simulink model "MPS_device_passive"  (R2018b)
settings: Solver=ode4  StartTime=0  StopTime=300  FixedStep=0.02  MaxStep=0.02  RelTol=1e-3  EnableMultiTasking=on
InitFcn:
  | %SSModel_calc
undefined symbols (not defined in the file): body, CentralPTOPreload, constraint, L, ML1Preload, ML2Preload, ML3Preload, ML4Preload, ML5Preload, ML6Preload, ML7Preload, ML8Preload, mrelative, pto, PTOrotation, SidePTO1Preload, SidePTO2Preload, SidePTO3Preload, SidePTO4Preload, simu, waves, X, Y, Z
libraries: nesl_utility x580, sm_lib x317, vrlib x72, WECSim_Lib x36
(part 19 of 27)

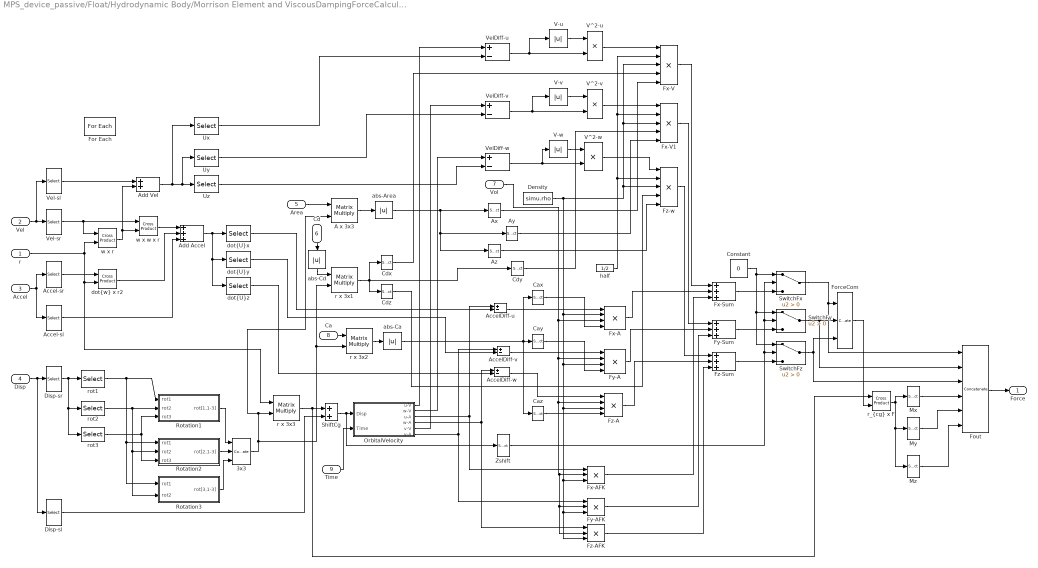
== system MPS_device_passive/Float/Hydrodynamic Body/Morrison Element and ViscousDampingForceCalculation/Morrison Element Variant Subsystem/Morrison Element On/Regular Wave Morison Force/MorrisonElements ==
  r : Inport  Partition=on  PartitionDimension=1  PartitionWidth=1  PartitionOffset=0
  Vel : Inport  Port=2
  Accel : Inport  Port=3
  Disp : Inport  Port=4
  Area : Inport  Port=5  Partition=on  PartitionDimension=1  PartitionWidth=1  PartitionOffset=0
  Cd : Inport  Port=6  Partition=on  PartitionDimension=1  PartitionWidth=1  PartitionOffset=0
  Vol : Inport  Port=7  Partition=on  PartitionDimension=1  PartitionWidth=1  PartitionOffset=0
  Ca : Inport  Port=8  Partition=on  PartitionDimension=1  PartitionWidth=1  PartitionOffset=0
  Time : Inport  Port=9
  3x3 : Concatenate  NumInputs=3  Mode=Multidimensional array
  A x 3x3 : Product  Multiplication=Matrix(*)
  Accel-sl : Selector  InputPortWidth=6  IndexOptions=Index vector (dialog)  Indices=[1 2 3]  OutputSizes=1
  Accel-sr : Selector  InputPortWidth=6  IndexOptions=Index vector (dialog)  Indices=[4 5 6]  OutputSizes=1
  AccelDiff-u : Sum  Inputs=+-
  AccelDiff-v : Sum  Inputs=+-
  AccelDiff-w : Sum  Inputs=+-
  Add Accel : Sum  Inputs=+++
  Add Vel : Sum
  Ax : Selector  InputPortWidth=3  IndexOptions=Index vector (dialog)  Indices=[1]  OutputSizes=1
  Ay : Selector  InputPortWidth=3  IndexOptions=Index vector (dialog)  Indices=[2]  OutputSizes=1
  Az : Selector  InputPortWidth=3  IndexOptions=Index vector (dialog)  Indices=[3]  OutputSizes=1
  Cax : Selector  InputPortWidth=3  IndexOptions=Index vector (dialog)  Indices=[1]  OutputSizes=1
  Cay : Selector  InputPortWidth=3  IndexOptions=Index vector (dialog)  Indices=[2]  OutputSizes=1
  Caz : Selector  InputPortWidth=3  IndexOptions=Index vector (dialog)  Indices=[3]  OutputSizes=1
  Cdx : Selector  InputPortWidth=3  IndexOptions=Index vector (dialog)  Indices=[1]  OutputSizes=1
  Cdy : Selector  InputPortWidth=3  IndexOptions=Index vector (dialog)  Indices=[2]  OutputSizes=1
  Cdz : Selector  InputPortWidth=3  IndexOptions=Index vector (dialog)  Indices=[3]  OutputSizes=1
  Constant : Constant  Value=0
  Density : Constant  Value=simu.rho
  Disp-sl : Selector  InputPortWidth=6  IndexOptions=Index vector (dialog)  Indices=[1 2 3]  OutputSizes=1
  Disp-sr : Selector  InputPortWidth=6  IndexOptions=Index vector (dialog)  Indices=[4 5 6]  OutputSizes=1
  For Each : ForEach  DisableCoverage=on  IndexMode=One-based
  ForceCom : Concatenate  NumInputs=3  ConcatenateDimension=2
  Fout : Concatenate  NumInputs=6  Mode=Multidimensional array  ConcatenateDimension=2
  Fx-A : Product  Inputs=4
  Fx-AFK : Product  Inputs=3
  Fx-Sum : Sum  Inputs=+++
  Fx-V : Product  Inputs=5
  Fx-V1 : Product  Inputs=5
  Fy-A : Product  Inputs=4
  Fy-AFK : Product  Inputs=3
  Fy-Sum : Sum  Inputs=+++
  Fz-A : Product  Inputs=4
  Fz-AFK : Product  Inputs=3
  Fz-Sum : Sum  Inputs=+++
  Fz-w : Product  Inputs=5
  Mx : Selector  InputPortWidth=3  IndexOptions=Index vector (dialog)  Indices=[1]  OutputSizes=1
  My : Selector  InputPortWidth=3  IndexOptions=Index vector (dialog)  Indices=[2]  OutputSizes=1
  Mz : Selector  InputPortWidth=3  IndexOptions=Index vector (dialog)  Indices=[3]  OutputSizes=1
  OrbitalVelocity : Subsystem
  Rotation1 : Subsystem
  Rotation2 : Subsystem
  Rotation3 : Subsystem
  ShiftCg : Sum
  SwitchFx : Switch  Criteria=u2 > Threshold
  SwitchFy : Switch  Criteria=u2 > Threshold
  SwitchFz : Switch  Criteria=u2 > Threshold
  Ux : Selector  InputPortWidth=3  IndexOptions=Index vector (dialog)  Indices=[1]  OutputSizes=1
  Uy : Selector  InputPortWidth=3  IndexOptions=Index vector (dialog)  Indices=[2]  OutputSizes=1
  Uz : Selector  InputPortWidth=3  IndexOptions=Index vector (dialog)  Indices=[3]  OutputSizes=1
  V-u : Abs
  V-v : Abs
  V-w : Abs
  V^2-u : Product
  V^2-v : Product
  V^2-w : Product
  Vel-sl : Selector  InputPortWidth=6  IndexOptions=Index vector (dialog)  Indices=[1 2 3]  OutputSizes=1
  "Vel-sr " : Selector  InputPortWidth=6  IndexOptions=Index vector (dialog)  Indices=[4 5 6]  OutputSizes=1
  VelDiff-u : Sum  Inputs=+-
  VelDiff-v : Sum  Inputs=+-
  VelDiff-w : Sum  Inputs=+-
  Zshift : Selector  InputPortWidth=3  IndexOptions=Index vector (dialog)  Indices=[3]  OutputSizes=1
  abs-Area : Abs
  abs-Ca : Abs
  abs-Cd : Abs
  "dot{U}x" : Selector  InputPortWidth=3  IndexOptions=Index vector (dialog)  Indices=[1]  OutputSizes=1
  "dot{U}y" : Selector  InputPortWidth=3  IndexOptions=Index vector (dialog)  Indices=[2]  OutputSizes=1
  "dot{U}z" : Selector  InputPortWidth=3  IndexOptions=Index vector (dialog)  Indices=[3]  OutputSizes=1
  "dot{w} x r2" : vrlib/Utilities/Cross Product
      settings: SourceProductBaseCode=VR
  half : Constant  Value=1/2
  r x 3x1 : Product  Multiplication=Matrix(*)
  r x 3x2 : Product  Multiplication=Matrix(*)
  r x 3x3 : Product  Multiplication=Matrix(*)
  "r_{cg} x F" : vrlib/Utilities/Cross Product
      settings: SourceProductBaseCode=VR
  rot1 : Selector  InputPortWidth=3  IndexOptions=Index vector (dialog)  Indices=[1]  OutputSizes=1
  rot2 : Selector  InputPortWidth=3  IndexOptions=Index vector (dialog)  Indices=[2]  OutputSizes=1
  rot3 : Selector  InputPortWidth=3  IndexOptions=Index vector (dialog)  Indices=[3]  OutputSizes=1
  w x r : vrlib/Utilities/Cross Product
      settings: SourceProductBaseCode=VR
  w x w x r : vrlib/Utilities/Cross Product
      settings: SourceProductBaseCode=VR
  Force : Outport  PortDimensions=[1 6]  ConcatenationDimension=1
  wires:
  Time/1 -> OrbitalVelocity/2(Time)
  abs-Cd/1 -> r x 3x1/1
  abs-Ca/1 -> Caz/1, Cay/1, Cax/1
  V-w/1 -> V^2-w/1
  Constant/1 -> SwitchFx/1, SwitchFz/1, SwitchFy/1
  Fx-V1/1 -> Fy-Sum/1
  Fy-A/1 -> Fy-Sum/2
  Cay/1 -> Fy-A/4
  AccelDiff-v/1 -> Fy-A/1
  Fy-AFK/1 -> Fy-Sum/3
  Fy-Sum/1 -> SwitchFy/3
  SwitchFy/1 -> ForceCom/2, Fout/2
  Cdy/1 -> Fx-V1/4
  Ay/1 -> Fx-V1/5
  OrbitalVelocity/5(v-V) -> VelDiff-v/1
  VelDiff-v/1 -> V^2-v/2, V-v/1
  V-v/1 -> V^2-v/1
  V^2-v/1 -> Fx-V1/1
  OrbitalVelocity/6(v-A) -> Fy-AFK/1, AccelDiff-v/1
  r x 3x2/1 -> abs-Ca/1
  Ca/1 -> r x 3x2/1
  r x 3x1/1 -> Cdx/1, Cdz/1, Cdy/1
  Cd/1 -> abs-Cd/1
  Cax/1 -> Fx-A/4
  Caz/1 -> Fz-A/4
  Fout/1 -> Force/1
  ForceCom/1 -> "r_{cg} x F"/2
  abs-Area/1 -> Ax/1, Az/1, Ay/1
  A x 3x3/1 -> abs-Area/1
  Cdz/1 -> Fz-w/4
  Cdx/1 -> Fx-V/4
  Ax/1 -> Fx-V/5
  Area/1 -> A x 3x3/1
  Az/1 -> Fz-w/5
  Fz-Sum/1 -> SwitchFz/3
  Fx-Sum/1 -> SwitchFx/3
  SwitchFx/1 -> ForceCom/1, Fout/1
  SwitchFz/1 -> Fout/3, ForceCom/3
  Zshift/1 -> SwitchFz/2, SwitchFx/2, SwitchFy/2
  VelDiff-u/1 -> V^2-u/2, V-u/1
  V-u/1 -> V^2-u/1
  3x3/1 -> r x 3x1/2, r x 3x2/2, r x 3x3/2, A x 3x3/2
  Mz/1 -> Fout/6
  My/1 -> Fout/5
  Mx/1 -> Fout/4
  "r_{cg} x F"/1 -> Mx/1, My/1, Mz/1
  Fz-AFK/1 -> Fz-Sum/3
  Fz-A/1 -> Fz-Sum/2
  Fz-w/1 -> Fz-Sum/1
  Fx-AFK/1 -> Fx-Sum/3
  Fx-A/1 -> Fx-Sum/2
  Fx-V/1 -> Fx-Sum/1
  OrbitalVelocity/4(w-A) -> AccelDiff-w/1, Fz-AFK/1
  AccelDiff-w/1 -> Fz-A/1
  Vol/1 -> Fx-A/3, Fz-A/2, Fx-AFK/2, Fz-AFK/2, Fy-AFK/2, Fy-A/2
  AccelDiff-u/1 -> Fx-A/1
  V^2-w/1 -> Fz-w/1
  Density/1 -> Fx-V/3, Fx-V1/3, Fz-w/3, Fx-A/2, Fz-A/3, Fx-AFK/3, Fz-AFK/3, Fy-AFK/3, Fy-A/3
  half/1 -> Fx-V/2, Fx-V1/2, Fz-w/2
  V^2-u/1 -> Fx-V/1
  VelDiff-w/1 -> V^2-w/2, V-w/1
  OrbitalVelocity/2(w-V) -> VelDiff-w/1
  OrbitalVelocity/1(u-V) -> VelDiff-u/1
  Uz/1 -> VelDiff-w/2
  Ux/1 -> VelDiff-u/2
  Uy/1 -> VelDiff-v/2
  Add Vel/1 -> Ux/1, Uz/1, Uy/1
  "dot{U}z"/1 -> AccelDiff-w/2
  OrbitalVelocity/3(u-A) -> Fx-AFK/1, AccelDiff-u/1
  "dot{U}x"/1 -> AccelDiff-u/2
  "dot{U}y"/1 -> AccelDiff-v/2
  ShiftCg/1 -> OrbitalVelocity/1(Disp), Zshift/1
  Disp-sl/1 -> ShiftCg/2
  r x 3x3/1 -> ShiftCg/1, "r_{cg} x F"/1
  Rotation3/1(rot[3,1-3]) -> 3x3/3
  Rotation1/1(rot[1,1-3]) -> 3x3/1
  Rotation2/1(rot[2,1-3]) -> 3x3/2
  rot2/1 -> Rotation1/2(rot2), Rotation2/2(rot2), Rotation3/2(rot2)
  rot1/1 -> Rotation1/1(rot1), Rotation2/1(rot1), Rotation3/1(rot1)
  rot3/1 -> Rotation1/3(rot3), Rotation2/3(rot3)
  Disp-sr/1 -> rot1/1, rot2/1, rot3/1
  Disp/1 -> Disp-sr/1, Disp-sl/1
  Vel-sl/1 -> Add Vel/1
  Add Accel/1 -> "dot{U}x"/1, "dot{U}y"/1, "dot{U}z"/1
  Accel-sl/1 -> Add Accel/3
  "dot{w} x r2"/1 -> Add Accel/2
  Accel-sr/1 -> "dot{w} x r2"/1
  Accel/1 -> Accel-sr/1, Accel-sl/1
  r/1 -> w x r/2, "dot{w} x r2"/2, r x 3x3/1
  "Vel-sr "/1 -> w x r/1, w x w x r/1
  w x w x r/1 -> Add Accel/1
  w x r/1 -> w x w x r/2, Add Vel/2
  Vel/1 -> "Vel-sr "/1, Vel-sl/1

== system MPS_device_passive/PTO P1F1/VisuP1F2/Hydrodynamic Body/Morrison Element and ViscousDampingForceCalculation/Morrison Element Variant Subsystem/Morrison Element On/Irregular Wave Morison Force ==
  displacement : Inport
  velocity : Inport  Port=2
  acceleration : Inport  Port=3
  time : Inport  Port=4
  Area : Constant  Value=body.morrisonElement.characteristicArea  VectorParams1D=off
  Ca : Constant  Value=body.morrisonElement.ca  VectorParams1D=off
  Cd : Constant  Value=body.morrisonElement.cd  VectorParams1D=off
  MESum : Sum  Inputs=+  CollapseMode=Specified dimension
  MorrisonElements : Subsystem  TreatAsAtomicUnit=on
  Reshape : Reshape
  Volume : Constant  Value=body.morrisonElement.VME  VectorParams1D=off
  "r_{g}" : Constant  Value=body.morrisonElement.rgME  VectorParams1D=off
  morison_force : Outport
  wires:
  time/1 -> MorrisonElements/9(Time)
  MESum/1 -> Reshape/1
  Reshape/1 -> morison_force/1
  MorrisonElements/1(Force) -> MESum/1
  Ca/1 -> MorrisonElements/8(Ca)
  Volume/1 -> MorrisonElements/7(Vol)
  acceleration/1 -> MorrisonElements/3(Accel)
  displacement/1 -> MorrisonElements/4(Disp)
  Cd/1 -> MorrisonElements/6(Cd)
  Area/1 -> MorrisonElements/5(A)
  "r_{g}"/1 -> MorrisonElements/1(r)
  velocity/1 -> MorrisonElements/2(Vel)

== system MPS_device_passive/PTO P1F1/VisuP1F2/Hydrodynamic Body/Morrison Element and ViscousDampingForceCalculation/Morrison Element Variant Subsystem/Morrison Element On/No Wave Morison Force ==
  displacement : Inport
  velocity : Inport  Port=2
  acceleration : Inport  Port=3
  time : Inport  Port=4
  Area : Constant  Value=body.morrisonElement.characteristicArea  VectorParams1D=off
  Ca : Constant  Value=body.morrisonElement.ca  VectorParams1D=off
  Cd : Constant  Value=body.morrisonElement.cd  VectorParams1D=off
  MESum : Sum  Inputs=+  CollapseMode=Specified dimension
  MorrisonElements : Subsystem  TreatAsAtomicUnit=on
  Reshape : Reshape
  Volume : Constant  Value=body.morrisonElement.VME  VectorParams1D=off
  "r_{g}" : Constant  Value=body.morrisonElement.rgME  VectorParams1D=off
  morison_force : Outport
  wires:
  time/1 -> MorrisonElements/9(Time)
  Reshape/1 -> morison_force/1
  MESum/1 -> Reshape/1
  acceleration/1 -> MorrisonElements/3(Accel)
  velocity/1 -> MorrisonElements/2(Vel)
  displacement/1 -> MorrisonElements/4(Disp)
  Ca/1 -> MorrisonElements/8(Ca)
  Volume/1 -> MorrisonElements/7(Vol)
  MorrisonElements/1(Force) -> MESum/1
  Cd/1 -> MorrisonElements/6(Cd)
  Area/1 -> MorrisonElements/5(Area)
  "r_{g}"/1 -> MorrisonElements/1(r)

== system MPS_device_passive/PTO P1F1/VisuP1F2/Hydrodynamic Body/Morrison Element and ViscousDampingForceCalculation/Morrison Element Variant Subsystem/Morrison Element On/Regular Wave Morison Force ==
  displacement : Inport
  velocity : Inport  Port=2
  acceleration : Inport  Port=3
  time : Inport  Port=4
  Area : Constant  Value=body.morrisonElement.characteristicArea  VectorParams1D=off
  Ca : Constant  Value=body.morrisonElement.ca  VectorParams1D=off
  Cd : Constant  Value=body.morrisonElement.cd  VectorParams1D=off
  MESum : Sum  Inputs=+  CollapseMode=Specified dimension
  MorrisonElements : Subsystem  TreatAsAtomicUnit=on
  Reshape : Reshape
  Volume : Constant  Value=body.morrisonElement.VME  VectorParams1D=off
  "r_{g}" : Constant  Value=body.morrisonElement.rgME  VectorParams1D=off
  morison_force : Outport
  wires:
  time/1 -> MorrisonElements/9(Time)
  Reshape/1 -> morison_force/1
  MESum/1 -> Reshape/1
  acceleration/1 -> MorrisonElements/3(Accel)
  velocity/1 -> MorrisonElements/2(Vel)
  displacement/1 -> MorrisonElements/4(Disp)
  Ca/1 -> MorrisonElements/8(Ca)
  Volume/1 -> MorrisonElements/7(Vol)
  MorrisonElements/1(Force) -> MESum/1
  Cd/1 -> MorrisonElements/6(Cd)
  Area/1 -> MorrisonElements/5(Area)
  "r_{g}"/1 -> MorrisonElements/1(r)

== system MPS_device_passive/PTO P2F2/VisuP2F3/Hydrodynamic Body/Morrison Element and ViscousDampingForceCalculation/Morrison Element Variant Subsystem/Morrison Element On/Irregular Wave Morison Force ==
  displacement : Inport
  velocity : Inport  Port=2
  acceleration : Inport  Port=3
  time : Inport  Port=4
  Area : Constant  Value=body.morrisonElement.characteristicArea  VectorParams1D=off
  Ca : Constant  Value=body.morrisonElement.ca  VectorParams1D=off
  Cd : Constant  Value=body.morrisonElement.cd  VectorParams1D=off
  MESum : Sum  Inputs=+  CollapseMode=Specified dimension
  MorrisonElements : Subsystem  TreatAsAtomicUnit=on
  Reshape : Reshape
  Volume : Constant  Value=body.morrisonElement.VME  VectorParams1D=off
  "r_{g}" : Constant  Value=body.morrisonElement.rgME  VectorParams1D=off
  morison_force : Outport
  wires:
  time/1 -> MorrisonElements/9(Time)
  MESum/1 -> Reshape/1
  Reshape/1 -> morison_force/1
  MorrisonElements/1(Force) -> MESum/1
  Ca/1 -> MorrisonElements/8(Ca)
  Volume/1 -> MorrisonElements/7(Vol)
  acceleration/1 -> MorrisonElements/3(Accel)
  displacement/1 -> MorrisonElements/4(Disp)
  Cd/1 -> MorrisonElements/6(Cd)
  Area/1 -> MorrisonElements/5(A)
  "r_{g}"/1 -> MorrisonElements/1(r)
  velocity/1 -> MorrisonElements/2(Vel)

== system MPS_device_passive/PTO P2F2/VisuP2F3/Hydrodynamic Body/Morrison Element and ViscousDampingForceCalculation/Morrison Element Variant Subsystem/Morrison Element On/No Wave Morison Force ==
  displacement : Inport
  velocity : Inport  Port=2
  acceleration : Inport  Port=3
  time : Inport  Port=4
  Area : Constant  Value=body.morrisonElement.characteristicArea  VectorParams1D=off
  Ca : Constant  Value=body.morrisonElement.ca  VectorParams1D=off
  Cd : Constant  Value=body.morrisonElement.cd  VectorParams1D=off
  MESum : Sum  Inputs=+  CollapseMode=Specified dimension
  MorrisonElements : Subsystem  TreatAsAtomicUnit=on
  Reshape : Reshape
  Volume : Constant  Value=body.morrisonElement.VME  VectorParams1D=off
  "r_{g}" : Constant  Value=body.morrisonElement.rgME  VectorParams1D=off
  morison_force : Outport
  wires:
  time/1 -> MorrisonElements/9(Time)
  Reshape/1 -> morison_force/1
  MESum/1 -> Reshape/1
  acceleration/1 -> MorrisonElements/3(Accel)
  velocity/1 -> MorrisonElements/2(Vel)
  displacement/1 -> MorrisonElements/4(Disp)
  Ca/1 -> MorrisonElements/8(Ca)
  Volume/1 -> MorrisonElements/7(Vol)
  MorrisonElements/1(Force) -> MESum/1
  Cd/1 -> MorrisonElements/6(Cd)
  Area/1 -> MorrisonElements/5(Area)
  "r_{g}"/1 -> MorrisonElements/1(r)

== system MPS_device_passive/PTO P2F2/VisuP2F3/Hydrodynamic Body/Morrison Element and ViscousDampingForceCalculation/Morrison Element Variant Subsystem/Morrison Element On/Regular Wave Morison Force ==
  displacement : Inport
  velocity : Inport  Port=2
  acceleration : Inport  Port=3
  time : Inport  Port=4
  Area : Constant  Value=body.morrisonElement.characteristicArea  VectorParams1D=off
  Ca : Constant  Value=body.morrisonElement.ca  VectorParams1D=off
  Cd : Constant  Value=body.morrisonElement.cd  VectorParams1D=off
  MESum : Sum  Inputs=+  CollapseMode=Specified dimension
  MorrisonElements : Subsystem  TreatAsAtomicUnit=on
  Reshape : Reshape
  Volume : Constant  Value=body.morrisonElement.VME  VectorParams1D=off
  "r_{g}" : Constant  Value=body.morrisonElement.rgME  VectorParams1D=off
  morison_force : Outport
  wires:
  time/1 -> MorrisonElements/9(Time)
  Reshape/1 -> morison_force/1
  MESum/1 -> Reshape/1
  acceleration/1 -> MorrisonElements/3(Accel)
  velocity/1 -> MorrisonElements/2(Vel)
  displacement/1 -> MorrisonElements/4(Disp)
  Ca/1 -> MorrisonElements/8(Ca)
  Volume/1 -> MorrisonElements/7(Vol)
  MorrisonElements/1(Force) -> MESum/1
  Cd/1 -> MorrisonElements/6(Cd)
  Area/1 -> MorrisonElements/5(Area)
  "r_{g}"/1 -> MorrisonElements/1(r)

== system MPS_device_passive/PTO P3F3/VisuP3F2/Hydrodynamic Body/Morrison Element and ViscousDampingForceCalculation/Morrison Element Variant Subsystem/Morrison Element On/Irregular Wave Morison Force ==
  displacement : Inport
  velocity : Inport  Port=2
  acceleration : Inport  Port=3
  time : Inport  Port=4
  Area : Constant  Value=body.morrisonElement.characteristicArea  VectorParams1D=off
  Ca : Constant  Value=body.morrisonElement.ca  VectorParams1D=off
  Cd : Constant  Value=body.morrisonElement.cd  VectorParams1D=off
  MESum : Sum  Inputs=+  CollapseMode=Specified dimension
  MorrisonElements : Subsystem  TreatAsAtomicUnit=on
  Reshape : Reshape
  Volume : Constant  Value=body.morrisonElement.VME  VectorParams1D=off
  "r_{g}" : Constant  Value=body.morrisonElement.rgME  VectorParams1D=off
  morison_force : Outport
  wires:
  time/1 -> MorrisonElements/9(Time)
  MESum/1 -> Reshape/1
  Reshape/1 -> morison_force/1
  MorrisonElements/1(Force) -> MESum/1
  Ca/1 -> MorrisonElements/8(Ca)
  Volume/1 -> MorrisonElements/7(Vol)
  acceleration/1 -> MorrisonElements/3(Accel)
  displacement/1 -> MorrisonElements/4(Disp)
  Cd/1 -> MorrisonElements/6(Cd)
  Area/1 -> MorrisonElements/5(A)
  "r_{g}"/1 -> MorrisonElements/1(r)
  velocity/1 -> MorrisonElements/2(Vel)

== system MPS_device_passive/PTO P3F3/VisuP3F2/Hydrodynamic Body/Morrison Element and ViscousDampingForceCalculation/Morrison Element Variant Subsystem/Morrison Element On/No Wave Morison Force ==
  displacement : Inport
  velocity : Inport  Port=2
  acceleration : Inport  Port=3
  time : Inport  Port=4
  Area : Constant  Value=body.morrisonElement.characteristicArea  VectorParams1D=off
  Ca : Constant  Value=body.morrisonElement.ca  VectorParams1D=off
  Cd : Constant  Value=body.morrisonElement.cd  VectorParams1D=off
  MESum : Sum  Inputs=+  CollapseMode=Specified dimension
  MorrisonElements : Subsystem  TreatAsAtomicUnit=on
  Reshape : Reshape
  Volume : Constant  Value=body.morrisonElement.VME  VectorParams1D=off
  "r_{g}" : Constant  Value=body.morrisonElement.rgME  VectorParams1D=off
  morison_force : Outport
  wires:
  time/1 -> MorrisonElements/9(Time)
  Reshape/1 -> morison_force/1
  MESum/1 -> Reshape/1
  acceleration/1 -> MorrisonElements/3(Accel)
  velocity/1 -> MorrisonElements/2(Vel)
  displacement/1 -> MorrisonElements/4(Disp)
  Ca/1 -> MorrisonElements/8(Ca)
  Volume/1 -> MorrisonElements/7(Vol)
  MorrisonElements/1(Force) -> MESum/1
  Cd/1 -> MorrisonElements/6(Cd)
  Area/1 -> MorrisonElements/5(Area)
  "r_{g}"/1 -> MorrisonElements/1(r)

== system MPS_device_passive/PTO P3F3/VisuP3F2/Hydrodynamic Body/Morrison Element and ViscousDampingForceCalculation/Morrison Element Variant Subsystem/Morrison Element On/Regular Wave Morison Force ==
  displacement : Inport
  velocity : Inport  Port=2
  acceleration : Inport  Port=3
  time : Inport  Port=4
  Area : Constant  Value=body.morrisonElement.characteristicArea  VectorParams1D=off
  Ca : Constant  Value=body.morrisonElement.ca  VectorParams1D=off
  Cd : Constant  Value=body.morrisonElement.cd  VectorParams1D=off
  MESum : Sum  Inputs=+  CollapseMode=Specified dimension
  MorrisonElements : Subsystem  TreatAsAtomicUnit=on
  Reshape : Reshape
  Volume : Constant  Value=body.morrisonElement.VME  VectorParams1D=off
  "r_{g}" : Constant  Value=body.morrisonElement.rgME  VectorParams1D=off
  morison_force : Outport
  wires:
  time/1 -> MorrisonElements/9(Time)
  Reshape/1 -> morison_force/1
  MESum/1 -> Reshape/1
  acceleration/1 -> MorrisonElements/3(Accel)
  velocity/1 -> MorrisonElements/2(Vel)
  displacement/1 -> MorrisonElements/4(Disp)
  Ca/1 -> MorrisonElements/8(Ca)
  Volume/1 -> MorrisonElements/7(Vol)
  MorrisonElements/1(Force) -> MESum/1
  Cd/1 -> MorrisonElements/6(Cd)
  Area/1 -> MorrisonElements/5(Area)
  "r_{g}"/1 -> MorrisonElements/1(r)

== system MPS_device_passive/PTO P4F4/VisuP4F1/Hydrodynamic Body/Morrison Element and ViscousDampingForceCalculation/Morrison Element Variant Subsystem/Morrison Element On/Irregular Wave Morison Force ==
  displacement : Inport
  velocity : Inport  Port=2
  acceleration : Inport  Port=3
  time : Inport  Port=4
  Area : Constant  Value=body.morrisonElement.characteristicArea  VectorParams1D=off
  Ca : Constant  Value=body.morrisonElement.ca  VectorParams1D=off
  Cd : Constant  Value=body.morrisonElement.cd  VectorParams1D=off
  MESum : Sum  Inputs=+  CollapseMode=Specified dimension
  MorrisonElements : Subsystem  TreatAsAtomicUnit=on
  Reshape : Reshape
  Volume : Constant  Value=body.morrisonElement.VME  VectorParams1D=off
  "r_{g}" : Constant  Value=body.morrisonElement.rgME  VectorParams1D=off
  morison_force : Outport
  wires:
  time/1 -> MorrisonElements/9(Time)
  MESum/1 -> Reshape/1
  Reshape/1 -> morison_force/1
  MorrisonElements/1(Force) -> MESum/1
  Ca/1 -> MorrisonElements/8(Ca)
  Volume/1 -> MorrisonElements/7(Vol)
  acceleration/1 -> MorrisonElements/3(Accel)
  displacement/1 -> MorrisonElements/4(Disp)
  Cd/1 -> MorrisonElements/6(Cd)
  Area/1 -> MorrisonElements/5(A)
  "r_{g}"/1 -> MorrisonElements/1(r)
  velocity/1 -> MorrisonElements/2(Vel)

== system MPS_device_passive/PTO P4F4/VisuP4F1/Hydrodynamic Body/Morrison Element and ViscousDampingForceCalculation/Morrison Element Variant Subsystem/Morrison Element On/No Wave Morison Force ==
  displacement : Inport
  velocity : Inport  Port=2
  acceleration : Inport  Port=3
  time : Inport  Port=4
  Area : Constant  Value=body.morrisonElement.characteristicArea  VectorParams1D=off
  Ca : Constant  Value=body.morrisonElement.ca  VectorParams1D=off
  Cd : Constant  Value=body.morrisonElement.cd  VectorParams1D=off
  MESum : Sum  Inputs=+  CollapseMode=Specified dimension
  MorrisonElements : Subsystem  TreatAsAtomicUnit=on
  Reshape : Reshape
  Volume : Constant  Value=body.morrisonElement.VME  VectorParams1D=off
  "r_{g}" : Constant  Value=body.morrisonElement.rgME  VectorParams1D=off
  morison_force : Outport
  wires:
  time/1 -> MorrisonElements/9(Time)
  Reshape/1 -> morison_force/1
  MESum/1 -> Reshape/1
  acceleration/1 -> MorrisonElements/3(Accel)
  velocity/1 -> MorrisonElements/2(Vel)
  displacement/1 -> MorrisonElements/4(Disp)
  Ca/1 -> MorrisonElements/8(Ca)
  Volume/1 -> MorrisonElements/7(Vol)
  MorrisonElements/1(Force) -> MESum/1
  Cd/1 -> MorrisonElements/6(Cd)
  Area/1 -> MorrisonElements/5(Area)
  "r_{g}"/1 -> MorrisonElements/1(r)

== system MPS_device_passive/PTO P4F4/VisuP4F1/Hydrodynamic Body/Morrison Element and ViscousDampingForceCalculation/Morrison Element Variant Subsystem/Morrison Element On/Regular Wave Morison Force ==
  displacement : Inport
  velocity : Inport  Port=2
  acceleration : Inport  Port=3
  time : Inport  Port=4
  Area : Constant  Value=body.morrisonElement.characteristicArea  VectorParams1D=off
  Ca : Constant  Value=body.morrisonElement.ca  VectorParams1D=off
  Cd : Constant  Value=body.morrisonElement.cd  VectorParams1D=off
  MESum : Sum  Inputs=+  CollapseMode=Specified dimension
  MorrisonElements : Subsystem  TreatAsAtomicUnit=on
  Reshape : Reshape
  Volume : Constant  Value=body.morrisonElement.VME  VectorParams1D=off
  "r_{g}" : Constant  Value=body.morrisonElement.rgME  VectorParams1D=off
  morison_force : Outport
  wires:
  time/1 -> MorrisonElements/9(Time)
  Reshape/1 -> morison_force/1
  MESum/1 -> Reshape/1
  acceleration/1 -> MorrisonElements/3(Accel)
  velocity/1 -> MorrisonElements/2(Vel)
  displacement/1 -> MorrisonElements/4(Disp)
  Ca/1 -> MorrisonElements/8(Ca)
  Volume/1 -> MorrisonElements/7(Vol)
  MorrisonElements/1(Force) -> MESum/1
  Cd/1 -> MorrisonElements/6(Cd)
  Area/1 -> MorrisonElements/5(Area)
  "r_{g}"/1 -> MorrisonElements/1(r)

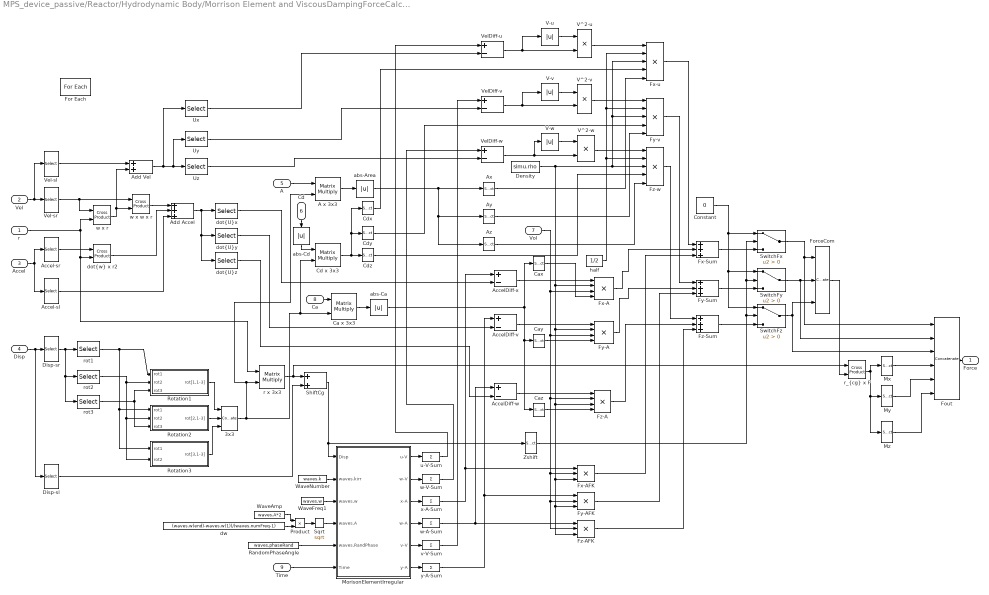
== system MPS_device_passive/Reactor/Hydrodynamic Body/Morrison Element and ViscousDampingForceCalculation/Morrison Element Variant Subsystem/Morrison Element On/Irregular Wave Excitation Force/MorrisonElements ==
  r : Inport  Partition=on  PartitionDimension=1  PartitionWidth=1  PartitionOffset=0
  Vel : Inport  Port=2
  Accel : Inport  Port=3
  Disp : Inport  Port=4
  A : Inport  Port=5  Partition=on  PartitionDimension=1  PartitionWidth=1  PartitionOffset=0
  Cd : Inport  Port=6  Partition=on  PartitionDimension=1  PartitionWidth=1  PartitionOffset=0
  Vol : Inport  Port=7  Partition=on  PartitionDimension=1  PartitionWidth=1  PartitionOffset=0
  Ca : Inport  Port=8  Partition=on  PartitionDimension=1  PartitionWidth=1  PartitionOffset=0
  Time : Inport  Port=9
  3x3 : Concatenate  NumInputs=3  Mode=Multidimensional array
  A x 3x3 : Product  Multiplication=Matrix(*)
  Accel-sl : Selector  InputPortWidth=6  IndexOptions=Index vector (dialog)  Indices=[1 2 3]  OutputSizes=1
  Accel-sr : Selector  InputPortWidth=6  IndexOptions=Index vector (dialog)  Indices=[4 5 6]  OutputSizes=1
  AccelDiff-v : Sum  Inputs=+-
  AccelDiff-w : Sum  Inputs=+-
  AccelDiff-x : Sum  Inputs=+-
  Add Accel : Sum  Inputs=+++
  Add Vel : Sum
  Ax : Selector  InputPortWidth=3  IndexOptions=Index vector (dialog)  Indices=[1]  OutputSizes=1
  Ay : Selector  InputPortWidth=3  IndexOptions=Index vector (dialog)  Indices=[2]  OutputSizes=1
  Az : Selector  InputPortWidth=3  IndexOptions=Index vector (dialog)  Indices=[3]  OutputSizes=1
  Ca x 3x3 : Product  Multiplication=Matrix(*)
  Cax : Selector  InputPortWidth=3  IndexOptions=Index vector (dialog)  Indices=[1]  OutputSizes=1
  Cay : Selector  InputPortWidth=3  IndexOptions=Index vector (dialog)  Indices=[2]  OutputSizes=1
  Caz : Selector  InputPortWidth=3  IndexOptions=Index vector (dialog)  Indices=[3]  OutputSizes=1
  Cd x 3x3 : Product  Multiplication=Matrix(*)
  Cdx : Selector  InputPortWidth=3  IndexOptions=Index vector (dialog)  Indices=[1]  OutputSizes=1
  Cdy : Selector  InputPortWidth=3  IndexOptions=Index vector (dialog)  Indices=[2]  OutputSizes=1
  Cdz : Selector  InputPortWidth=3  IndexOptions=Index vector (dialog)  Indices=[3]  OutputSizes=1
  Constant : Constant  Value=0
  Density : Constant  Value=simu.rho
  Disp-sl : Selector  InputPortWidth=6  IndexOptions=Index vector (dialog)  Indices=[1 2 3]  OutputSizes=1
  Disp-sr : Selector  InputPortWidth=6  IndexOptions=Index vector (dialog)  Indices=[4 5 6]  OutputSizes=1
  For Each : ForEach  DisableCoverage=on  IndexMode=One-based
  ForceCom : Concatenate  NumInputs=3  ConcatenateDimension=2
  Fout : Concatenate  NumInputs=6  Mode=Multidimensional array  ConcatenateDimension=2
  Fx-A : Product  Inputs=4
  Fx-AFK : Product  Inputs=3
  Fx-Sum : Sum  Inputs=+++
  Fx-u : Product  Inputs=5
  Fy-A : Product  Inputs=4
  Fy-AFK : Product  Inputs=3
  Fy-Sum : Sum  Inputs=+++
  Fy-v : Product  Inputs=5
  Fz-A : Product  Inputs=4
  Fz-AFK : Product  Inputs=3
  Fz-Sum : Sum  Inputs=+++
  Fz-w : Product  Inputs=5
  MorisonElementIrregular : Subsystem  TreatAsAtomicUnit=on
  Mx : Selector  InputPortWidth=3  IndexOptions=Index vector (dialog)  Indices=[1]  OutputSizes=1
  My : Selector  InputPortWidth=3  IndexOptions=Index vector (dialog)  Indices=[2]  OutputSizes=1
  Mz : Selector  InputPortWidth=3  IndexOptions=Index vector (dialog)  Indices=[3]  OutputSizes=1
  Product : Product
  RandomPhaseAngle : Constant  Value=waves.phaseRand  VectorParams1D=off
  Rotation1 : Subsystem
  Rotation2 : Subsystem
  Rotation3 : Subsystem
  ShiftCg : Sum
  Sqrt : Sqrt  SaturateOnIntegerOverflow=on
  SwitchFx : Switch  Criteria=u2 > Threshold
  SwitchFy : Switch  Criteria=u2 > Threshold
  SwitchFz : Switch  Criteria=u2 > Threshold
  Ux : Selector  InputPortWidth=3  IndexOptions=Index vector (dialog)  Indices=[1]  OutputSizes=1
  Uy : Selector  InputPortWidth=3  IndexOptions=Index vector (dialog)  Indices=[2]  OutputSizes=1
  Uz : Selector  InputPortWidth=3  IndexOptions=Index vector (dialog)  Indices=[3]  OutputSizes=1
  V-u : Abs
  V-v : Abs
  V-w : Abs
  V^2-u : Product
  V^2-v : Product
  V^2-w : Product
  Vel-sl : Selector  InputPortWidth=6  IndexOptions=Index vector (dialog)  Indices=[1 2 3]  OutputSizes=1
  "Vel-sr " : Selector  InputPortWidth=6  IndexOptions=Index vector (dialog)  Indices=[4 5 6]  OutputSizes=1
  VelDiff-u : Sum  Inputs=+-
  VelDiff-v : Sum  Inputs=+-
  VelDiff-w : Sum  Inputs=+-
  WaveAmp : Constant  Value=waves.A*2  VectorParams1D=off
  WaveFreq1 : Constant  Value=waves.w  VectorParams1D=off
  WaveNumber : Constant  Value=waves.k  VectorParams1D=off
  Zshift : Selector  InputPortWidth=3  IndexOptions=Index vector (dialog)  Indices=[3]  OutputSizes=1
  abs-Area : Abs
  abs-Ca : Abs
  abs-Cd : Abs
  "dot{U}x" : Selector  InputPortWidth=3  IndexOptions=Index vector (dialog)  Indices=[1]  OutputSizes=1
  "dot{U}y" : Selector  InputPortWidth=3  IndexOptions=Index vector (dialog)  Indices=[2]  OutputSizes=1
  "dot{U}z" : Selector  InputPortWidth=3  IndexOptions=Index vector (dialog)  Indices=[3]  OutputSizes=1
  "dot{w} x r2" : vrlib/Utilities/Cross Product
      settings: SourceProductBaseCode=VR
  dw : Constant  Value=(waves.w(end)-waves.w(1))/(waves.numFreq-1)  VectorParams1D=off
  half : Constant  Value=1/2
  r x 3x3 : Product  Multiplication=Matrix(*)
  "r_{cg} x F" : vrlib/Utilities/Cross Product
      settings: SourceProductBaseCode=VR
  rot1 : Selector  InputPortWidth=3  IndexOptions=Index vector (dialog)  Indices=[1]  OutputSizes=1
  rot2 : Selector  InputPortWidth=3  IndexOptions=Index vector (dialog)  Indices=[2]  OutputSizes=1
  rot3 : Selector  InputPortWidth=3  IndexOptions=Index vector (dialog)  Indices=[3]  OutputSizes=1
  u-V-Sum : Sum  Inputs=+  CollapseMode=Specified dimension
  v-V-Sum : Sum  Inputs=+  CollapseMode=Specified dimension
  w x r : vrlib/Utilities/Cross Product
      settings: SourceProductBaseCode=VR
  w x w x r : vrlib/Utilities/Cross Product
      settings: SourceProductBaseCode=VR
  w-A-Sum : Sum  Inputs=+  CollapseMode=Specified dimension
  w-V-Sum : Sum  Inputs=+  CollapseMode=Specified dimension
  x-A-Sum : Sum  Inputs=+  CollapseMode=Specified dimension
  y-A-Sum : Sum  Inputs=+  CollapseMode=Specified dimension
  Force : Outport  PortDimensions=[1 6]  ConcatenationDimension=1
  wires:
  Time/1 -> MorisonElementIrregular/6(Time)
  abs-Cd/1 -> Cd x 3x3/1
  abs-Ca/1 -> Cay/1, Caz/1, Cax/1
  Fy-AFK/1 -> Fy-Sum/3
  Fy-A/1 -> Fy-Sum/2
  AccelDiff-v/1 -> Fy-A/1
  Cay/1 -> Fy-A/4
  y-A-Sum/1 -> AccelDiff-v/1, Fy-AFK/1
  Fy-v/1 -> Fy-Sum/1
  Fy-Sum/1 -> SwitchFy/3
  SwitchFy/1 -> ForceCom/2, Fout/2
  Cdy/1 -> Fy-v/4
  Ay/1 -> Fy-v/5
  V^2-v/1 -> Fy-v/1
  v-V-Sum/1 -> VelDiff-v/1
  V-v/1 -> V^2-v/1
  VelDiff-v/1 -> V^2-v/2, V-v/1
  V-w/1 -> V^2-w/1
  MorisonElementIrregular/6(y-A) -> y-A-Sum/1
  MorisonElementIrregular/5(v-V) -> v-V-Sum/1
  V-u/1 -> V^2-u/1
  MorisonElementIrregular/4(w-A) -> w-A-Sum/1
  MorisonElementIrregular/3(x-A) -> x-A-Sum/1
  MorisonElementIrregular/2(w-V) -> w-V-Sum/1
  Sqrt/1 -> MorisonElementIrregular/4(waves.A)
  Product/1 -> Sqrt/1
  dw/1 -> Product/2
  WaveAmp/1 -> Product/1
  MorisonElementIrregular/1(u-V) -> u-V-Sum/1
  RandomPhaseAngle/1 -> MorisonElementIrregular/5(waves.RandPhase)
  WaveFreq1/1 -> MorisonElementIrregular/3(waves.w)
  WaveNumber/1 -> MorisonElementIrregular/2(waves.kirr)
  Ca x 3x3/1 -> abs-Ca/1
  Ca/1 -> Ca x 3x3/1
  Cd x 3x3/1 -> Cdx/1, Cdy/1, Cdz/1
  Cd/1 -> abs-Cd/1
  Cax/1 -> Fx-A/4
  Caz/1 -> Fz-A/4
  Fout/1 -> Force/1
  ForceCom/1 -> "r_{cg} x F"/2
  abs-Area/1 -> Ax/1, Az/1, Ay/1
  A x 3x3/1 -> abs-Area/1
  Cdz/1 -> Fz-w/4
  Cdx/1 -> Fx-u/4
  Ax/1 -> Fx-u/5
  A/1 -> A x 3x3/1
  Az/1 -> Fz-w/5
  Fz-Sum/1 -> SwitchFz/3
  Fx-Sum/1 -> SwitchFx/3
  SwitchFx/1 -> ForceCom/1, Fout/1
  SwitchFz/1 -> Fout/3, ForceCom/3
  Zshift/1 -> SwitchFz/2, SwitchFx/2, SwitchFy/2
  VelDiff-u/1 -> V^2-u/2, V-u/1
  3x3/1 -> Cd x 3x3/2, Ca x 3x3/2, r x 3x3/2, A x 3x3/2
  Mz/1 -> Fout/6
  My/1 -> Fout/5
  Mx/1 -> Fout/4
  "r_{cg} x F"/1 -> Mx/1, My/1, Mz/1
  Constant/1 -> SwitchFx/1, SwitchFz/1, SwitchFy/1
  Fz-AFK/1 -> Fz-Sum/3
  Fz-A/1 -> Fz-Sum/2
  Fz-w/1 -> Fz-Sum/1
  Fx-AFK/1 -> Fx-Sum/3
  Fx-A/1 -> Fx-Sum/2
  Fx-u/1 -> Fx-Sum/1
  w-A-Sum/1 -> Fz-AFK/1, AccelDiff-w/1
  AccelDiff-w/1 -> Fz-A/1
  Vol/1 -> Fx-A/3, Fz-A/2, Fx-AFK/2, Fz-AFK/2, Fy-AFK/2, Fy-A/3
  AccelDiff-x/1 -> Fx-A/1
  V^2-w/1 -> Fz-w/1
  Density/1 -> Fz-w/3, Fx-u/3, Fy-v/3, Fx-A/2, Fz-A/3, Fx-AFK/3, Fz-AFK/3, Fy-AFK/3, Fy-A/2
  half/1 -> Fx-u/2, Fy-v/2, Fz-w/2
  V^2-u/1 -> Fx-u/1
  VelDiff-w/1 -> V-w/1, V^2-w/2
  w-V-Sum/1 -> VelDiff-w/1
  u-V-Sum/1 -> VelDiff-u/1
  Uz/1 -> VelDiff-w/2
  Ux/1 -> VelDiff-u/2
  Uy/1 -> VelDiff-v/2
  Add Vel/1 -> Uz/1, Uy/1, Ux/1
  "dot{U}z"/1 -> AccelDiff-w/2
  x-A-Sum/1 -> AccelDiff-x/1, Fx-AFK/1
  "dot{U}x"/1 -> AccelDiff-x/2
  "dot{U}y"/1 -> AccelDiff-v/2
  ShiftCg/1 -> Zshift/1, MorisonElementIrregular/1(Disp)
  Disp-sl/1 -> ShiftCg/2
  r x 3x3/1 -> ShiftCg/1, "r_{cg} x F"/1
  Rotation3/1(rot[3,1-3]) -> 3x3/3
  Rotation1/1(rot[1,1-3]) -> 3x3/1
  Rotation2/1(rot[2,1-3]) -> 3x3/2
  rot2/1 -> Rotation1/2(rot2), Rotation2/2(rot2), Rotation3/2(rot2)
  rot1/1 -> Rotation1/1(rot1), Rotation2/1(rot1), Rotation3/1(rot1)
  rot3/1 -> Rotation1/3(rot3), Rotation2/3(rot3)
  Disp-sr/1 -> rot1/1, rot2/1, rot3/1
  Disp/1 -> Disp-sr/1, Disp-sl/1
  Vel-sl/1 -> Add Vel/1
  Add Accel/1 -> "dot{U}x"/1, "dot{U}y"/1, "dot{U}z"/1
  Accel-sl/1 -> Add Accel/3
  "dot{w} x r2"/1 -> Add Accel/2
  Accel-sr/1 -> "dot{w} x r2"/1
  Accel/1 -> Accel-sr/1, Accel-sl/1
  r/1 -> w x r/2, "dot{w} x r2"/2, r x 3x3/1
  "Vel-sr "/1 -> w x r/1, w x w x r/1
  w x w x r/1 -> Add Accel/1
  w x r/1 -> w x w x r/2, Add Vel/2
  Vel/1 -> "Vel-sr "/1, Vel-sl/1

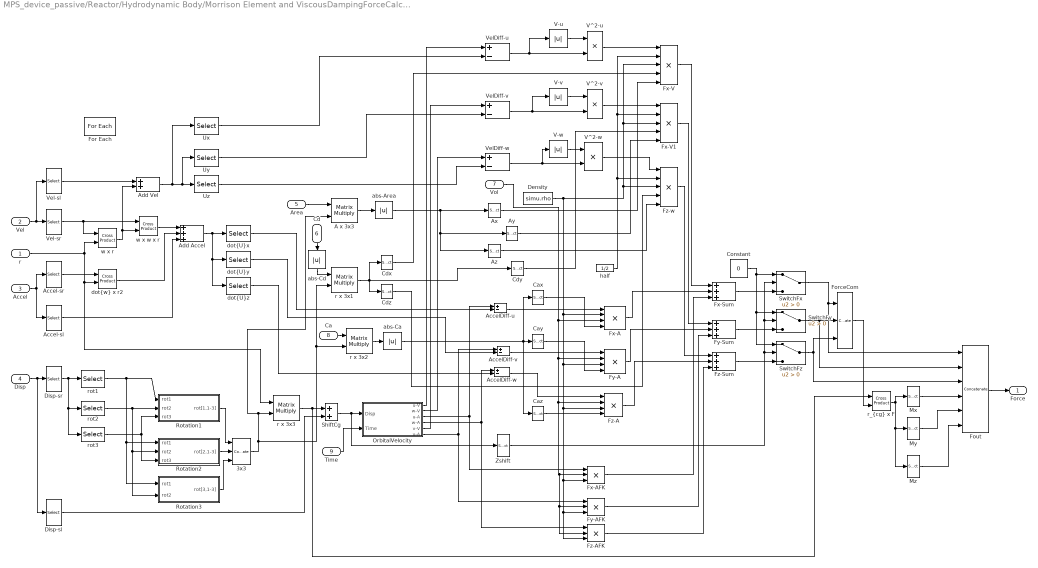
== system MPS_device_passive/Reactor/Hydrodynamic Body/Morrison Element and ViscousDampingForceCalculation/Morrison Element Variant Subsystem/Morrison Element On/No Wave Excitation Force/MorrisonElements ==
  r : Inport  Partition=on  PartitionDimension=1  PartitionWidth=1  PartitionOffset=0
  Vel : Inport  Port=2
  Accel : Inport  Port=3
  Disp : Inport  Port=4
  Area : Inport  Port=5  Partition=on  PartitionDimension=1  PartitionWidth=1  PartitionOffset=0
  Cd : Inport  Port=6  Partition=on  PartitionDimension=1  PartitionWidth=1  PartitionOffset=0
  Vol : Inport  Port=7  Partition=on  PartitionDimension=1  PartitionWidth=1  PartitionOffset=0
  Ca : Inport  Port=8  Partition=on  PartitionDimension=1  PartitionWidth=1  PartitionOffset=0
  Time : Inport  Port=9
  3x3 : Concatenate  NumInputs=3  Mode=Multidimensional array
  A x 3x3 : Product  Multiplication=Matrix(*)
  Accel-sl : Selector  InputPortWidth=6  IndexOptions=Index vector (dialog)  Indices=[1 2 3]  OutputSizes=1
  Accel-sr : Selector  InputPortWidth=6  IndexOptions=Index vector (dialog)  Indices=[4 5 6]  OutputSizes=1
  AccelDiff-u : Sum  Inputs=+-
  AccelDiff-v : Sum  Inputs=+-
  AccelDiff-w : Sum  Inputs=+-
  Add Accel : Sum  Inputs=+++
  Add Vel : Sum
  Ax : Selector  InputPortWidth=3  IndexOptions=Index vector (dialog)  Indices=[1]  OutputSizes=1
  Ay : Selector  InputPortWidth=3  IndexOptions=Index vector (dialog)  Indices=[2]  OutputSizes=1
  Az : Selector  InputPortWidth=3  IndexOptions=Index vector (dialog)  Indices=[3]  OutputSizes=1
  Cax : Selector  InputPortWidth=3  IndexOptions=Index vector (dialog)  Indices=[1]  OutputSizes=1
  Cay : Selector  InputPortWidth=3  IndexOptions=Index vector (dialog)  Indices=[2]  OutputSizes=1
  Caz : Selector  InputPortWidth=3  IndexOptions=Index vector (dialog)  Indices=[3]  OutputSizes=1
  Cdx : Selector  InputPortWidth=3  IndexOptions=Index vector (dialog)  Indices=[1]  OutputSizes=1
  Cdy : Selector  InputPortWidth=3  IndexOptions=Index vector (dialog)  Indices=[2]  OutputSizes=1
  Cdz : Selector  InputPortWidth=3  IndexOptions=Index vector (dialog)  Indices=[3]  OutputSizes=1
  Constant : Constant  Value=0
  Density : Constant  Value=simu.rho
  Disp-sl : Selector  InputPortWidth=6  IndexOptions=Index vector (dialog)  Indices=[1 2 3]  OutputSizes=1
  Disp-sr : Selector  InputPortWidth=6  IndexOptions=Index vector (dialog)  Indices=[4 5 6]  OutputSizes=1
  For Each : ForEach  DisableCoverage=on  IndexMode=One-based
  ForceCom : Concatenate  NumInputs=3  ConcatenateDimension=2
  Fout : Concatenate  NumInputs=6  Mode=Multidimensional array  ConcatenateDimension=2
  Fx-A : Product  Inputs=4
  Fx-AFK : Product  Inputs=3
  Fx-Sum : Sum  Inputs=+++
  Fx-V : Product  Inputs=5
  Fx-V1 : Product  Inputs=5
  Fy-A : Product  Inputs=4
  Fy-AFK : Product  Inputs=3
  Fy-Sum : Sum  Inputs=+++
  Fz-A : Product  Inputs=4
  Fz-AFK : Product  Inputs=3
  Fz-Sum : Sum  Inputs=+++
  Fz-w : Product  Inputs=5
  Mx : Selector  InputPortWidth=3  IndexOptions=Index vector (dialog)  Indices=[1]  OutputSizes=1
  My : Selector  InputPortWidth=3  IndexOptions=Index vector (dialog)  Indices=[2]  OutputSizes=1
  Mz : Selector  InputPortWidth=3  IndexOptions=Index vector (dialog)  Indices=[3]  OutputSizes=1
  OrbitalVelocity : Subsystem
  Rotation1 : Subsystem
  Rotation2 : Subsystem
  Rotation3 : Subsystem
  ShiftCg : Sum
  SwitchFx : Switch  Criteria=u2 > Threshold
  SwitchFy : Switch  Criteria=u2 > Threshold
  SwitchFz : Switch  Criteria=u2 > Threshold
  Ux : Selector  InputPortWidth=3  IndexOptions=Index vector (dialog)  Indices=[1]  OutputSizes=1
  Uy : Selector  InputPortWidth=3  IndexOptions=Index vector (dialog)  Indices=[2]  OutputSizes=1
  Uz : Selector  InputPortWidth=3  IndexOptions=Index vector (dialog)  Indices=[3]  OutputSizes=1
  V-u : Abs
  V-v : Abs
  V-w : Abs
  V^2-u : Product
  V^2-v : Product
  V^2-w : Product
  Vel-sl : Selector  InputPortWidth=6  IndexOptions=Index vector (dialog)  Indices=[1 2 3]  OutputSizes=1
  "Vel-sr " : Selector  InputPortWidth=6  IndexOptions=Index vector (dialog)  Indices=[4 5 6]  OutputSizes=1
  VelDiff-u : Sum  Inputs=+-
  VelDiff-v : Sum  Inputs=+-
  VelDiff-w : Sum  Inputs=+-
  Zshift : Selector  InputPortWidth=3  IndexOptions=Index vector (dialog)  Indices=[3]  OutputSizes=1
  abs-Area : Abs
  abs-Ca : Abs
  abs-Cd : Abs
  "dot{U}x" : Selector  InputPortWidth=3  IndexOptions=Index vector (dialog)  Indices=[1]  OutputSizes=1
  "dot{U}y" : Selector  InputPortWidth=3  IndexOptions=Index vector (dialog)  Indices=[2]  OutputSizes=1
  "dot{U}z" : Selector  InputPortWidth=3  IndexOptions=Index vector (dialog)  Indices=[3]  OutputSizes=1
  "dot{w} x r2" : vrlib/Utilities/Cross Product
      settings: SourceProductBaseCode=VR
  half : Constant  Value=1/2
  r x 3x1 : Product  Multiplication=Matrix(*)
  r x 3x2 : Product  Multiplication=Matrix(*)
  r x 3x3 : Product  Multiplication=Matrix(*)
  "r_{cg} x F" : vrlib/Utilities/Cross Product
      settings: SourceProductBaseCode=VR
  rot1 : Selector  InputPortWidth=3  IndexOptions=Index vector (dialog)  Indices=[1]  OutputSizes=1
  rot2 : Selector  InputPortWidth=3  IndexOptions=Index vector (dialog)  Indices=[2]  OutputSizes=1
  rot3 : Selector  InputPortWidth=3  IndexOptions=Index vector (dialog)  Indices=[3]  OutputSizes=1
  w x r : vrlib/Utilities/Cross Product
      settings: SourceProductBaseCode=VR
  w x w x r : vrlib/Utilities/Cross Product
      settings: SourceProductBaseCode=VR
  Force : Outport  PortDimensions=[1 6]  ConcatenationDimension=1
  wires:
  Time/1 -> OrbitalVelocity/2(Time)
  abs-Cd/1 -> r x 3x1/1
  abs-Ca/1 -> Caz/1, Cay/1, Cax/1
  V-w/1 -> V^2-w/1
  Constant/1 -> SwitchFx/1, SwitchFz/1, SwitchFy/1
  Fx-V1/1 -> Fy-Sum/1
  Fy-A/1 -> Fy-Sum/2
  Cay/1 -> Fy-A/4
  AccelDiff-v/1 -> Fy-A/1
  Fy-AFK/1 -> Fy-Sum/3
  Fy-Sum/1 -> SwitchFy/3
  SwitchFy/1 -> ForceCom/2, Fout/2
  Cdy/1 -> Fx-V1/4
  Ay/1 -> Fx-V1/5
  OrbitalVelocity/5(v-V) -> VelDiff-v/1
  VelDiff-v/1 -> V^2-v/2, V-v/1
  V-v/1 -> V^2-v/1
  V^2-v/1 -> Fx-V1/1
  OrbitalVelocity/6(v-A) -> Fy-AFK/1, AccelDiff-v/1
  r x 3x2/1 -> abs-Ca/1
  Ca/1 -> r x 3x2/1
  r x 3x1/1 -> Cdx/1, Cdz/1, Cdy/1
  Cd/1 -> abs-Cd/1
  Cax/1 -> Fx-A/4
  Caz/1 -> Fz-A/4
  Fout/1 -> Force/1
  ForceCom/1 -> "r_{cg} x F"/2
  abs-Area/1 -> Ax/1, Az/1, Ay/1
  A x 3x3/1 -> abs-Area/1
  Cdz/1 -> Fz-w/4
  Cdx/1 -> Fx-V/4
  Ax/1 -> Fx-V/5
  Area/1 -> A x 3x3/1
  Az/1 -> Fz-w/5
  Fz-Sum/1 -> SwitchFz/3
  Fx-Sum/1 -> SwitchFx/3
  SwitchFx/1 -> ForceCom/1, Fout/1
  SwitchFz/1 -> Fout/3, ForceCom/3
  Zshift/1 -> SwitchFz/2, SwitchFx/2, SwitchFy/2
  VelDiff-u/1 -> V^2-u/2, V-u/1
  V-u/1 -> V^2-u/1
  3x3/1 -> r x 3x1/2, r x 3x2/2, r x 3x3/2, A x 3x3/2
  Mz/1 -> Fout/6
  My/1 -> Fout/5
  Mx/1 -> Fout/4
  "r_{cg} x F"/1 -> Mx/1, My/1, Mz/1
  Fz-AFK/1 -> Fz-Sum/3
  Fz-A/1 -> Fz-Sum/2
  Fz-w/1 -> Fz-Sum/1
  Fx-AFK/1 -> Fx-Sum/3
  Fx-A/1 -> Fx-Sum/2
  Fx-V/1 -> Fx-Sum/1
  OrbitalVelocity/4(w-A) -> AccelDiff-w/1, Fz-AFK/1
  AccelDiff-w/1 -> Fz-A/1
  Vol/1 -> Fx-A/3, Fz-A/2, Fx-AFK/2, Fz-AFK/2, Fy-AFK/2, Fy-A/2
  AccelDiff-u/1 -> Fx-A/1
  V^2-w/1 -> Fz-w/1
  Density/1 -> Fx-V/3, Fx-V1/3, Fz-w/3, Fx-A/2, Fz-A/3, Fx-AFK/3, Fz-AFK/3, Fy-AFK/3, Fy-A/3
  half/1 -> Fx-V/2, Fx-V1/2, Fz-w/2
  V^2-u/1 -> Fx-V/1
  VelDiff-w/1 -> V^2-w/2, V-w/1
  OrbitalVelocity/2(w-V) -> VelDiff-w/1
  OrbitalVelocity/1(u-V) -> VelDiff-u/1
  Uz/1 -> VelDiff-w/2
  Ux/1 -> VelDiff-u/2
  Uy/1 -> VelDiff-v/2
  Add Vel/1 -> Ux/1, Uz/1, Uy/1
  "dot{U}z"/1 -> AccelDiff-w/2
  OrbitalVelocity/3(u-A) -> Fx-AFK/1, AccelDiff-u/1
  "dot{U}x"/1 -> AccelDiff-u/2
  "dot{U}y"/1 -> AccelDiff-v/2
  ShiftCg/1 -> OrbitalVelocity/1(Disp), Zshift/1
  Disp-sl/1 -> ShiftCg/2
  r x 3x3/1 -> ShiftCg/1, "r_{cg} x F"/1
  Rotation3/1(rot[3,1-3]) -> 3x3/3
  Rotation1/1(rot[1,1-3]) -> 3x3/1
  Rotation2/1(rot[2,1-3]) -> 3x3/2
  rot2/1 -> Rotation1/2(rot2), Rotation2/2(rot2), Rotation3/2(rot2)
  rot1/1 -> Rotation1/1(rot1), Rotation2/1(rot1), Rotation3/1(rot1)
  rot3/1 -> Rotation1/3(rot3), Rotation2/3(rot3)
  Disp-sr/1 -> rot1/1, rot2/1, rot3/1
  Disp/1 -> Disp-sr/1, Disp-sl/1
  Vel-sl/1 -> Add Vel/1
  Add Accel/1 -> "dot{U}x"/1, "dot{U}y"/1, "dot{U}z"/1
  Accel-sl/1 -> Add Accel/3
  "dot{w} x r2"/1 -> Add Accel/2
  Accel-sr/1 -> "dot{w} x r2"/1
  Accel/1 -> Accel-sr/1, Accel-sl/1
  r/1 -> w x r/2, "dot{w} x r2"/2, r x 3x3/1
  "Vel-sr "/1 -> w x r/1, w x w x r/1
  w x w x r/1 -> Add Accel/1
  w x r/1 -> w x w x r/2, Add Vel/2
  Vel/1 -> "Vel-sr "/1, Vel-sl/1
